simulink model "DEF_2SG"  (R2022b)
settings: Solver=FixedStepAuto  StartTime=0  StopTime=5  FixedStep=Ts  RelTol=1e-3
undefined symbols (not defined in the file or in its folder): ApparatusDiscreDamping, ApparatusPara, ApparatusPowerFlow, ApparatusType, OtherInputs, PowerFlow, Sbase, Ts, Vbase, Wbase, x_e, Ybase, Zbase
libraries: SimplusGT x6, spsGroundLib x5, spsThreePhaseSeriesRLCBranchLib x4, spsControlledCurrentSourceLib x3, spsCurrentMeasurementLib x3, spsVoltageMeasurementLib x3, spsThreePhaseParallelRLCBranchLib x2, spsabctoAlphaBetaZeroLib x2, spspowerguiLib x1
settings Model: Creator=yz34218  LastModifiedBy=yz34218

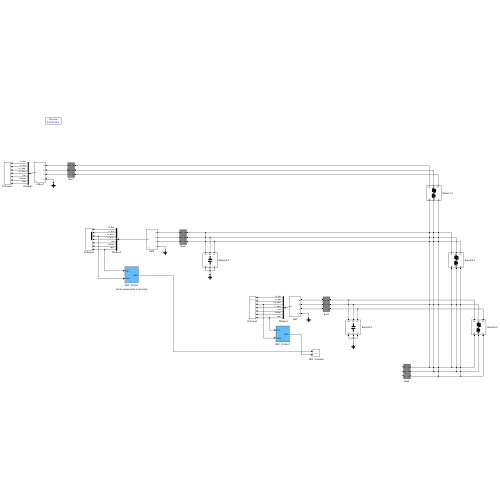
[thumbnail: Simulink's stored preview of the top-level diagram]
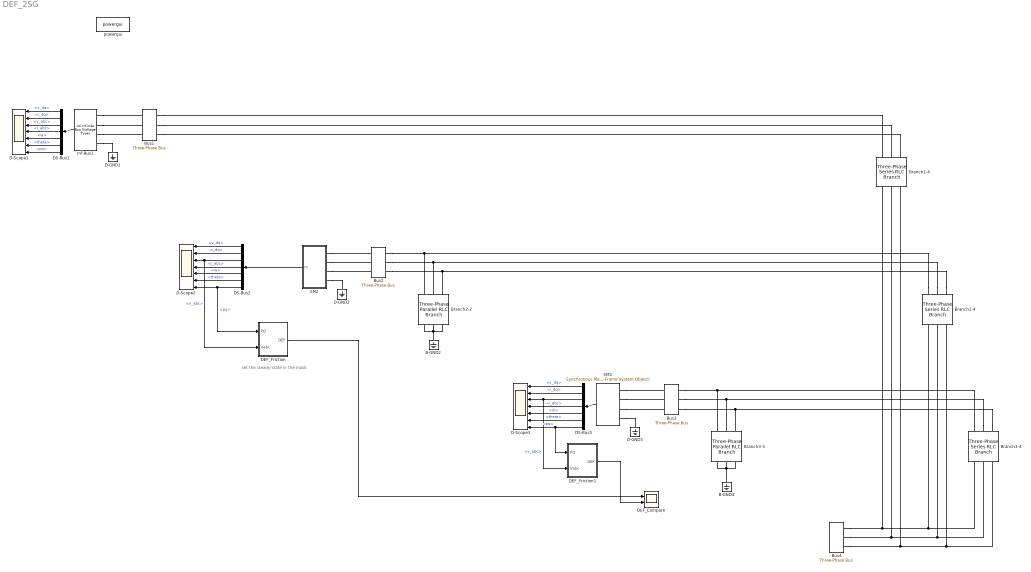
== system DEF_2SG ==
  note: set the steady-state in the mask
  B-GND2 : spsGroundLib/Ground  LConnTagsString=a
  B-GND4 : spsGroundLib/Ground  LConnTagsString=a
  Branch1-4 : spsThreePhaseSeriesRLCBranchLib/Three-Phase Series RLC Branch  LConnTagsString=A|B|C  RConnTagsString=A|B|C  BranchType=RL  Resistance=(0.1)*Zbase  Inductance=(1)*Zbase/Wbase  Capacitance=1e-6  Measurements=None
  Branch2-2 : spsThreePhaseParallelRLCBranchLib/Three-Phase Parallel RLC Branch  LConnTagsString=A|B|C  RConnTagsString=A|B|C  BranchType=C  Resistance=(Inf)*Zbase  Inductance=(Inf)*Zbase/Wbase  Capacitance=(0.3)*Ybase/Wbase  Measurements=None
  Branch2-4 : spsThreePhaseSeriesRLCBranchLib/Three-Phase Series RLC Branch  LConnTagsString=A|B|C  RConnTagsString=A|B|C  BranchType=RL  Resistance=(0.03)*Zbase  Inductance=(0.3)*Zbase/Wbase  Capacitance=1e-6  Measurements=None
  Branch3-3 : spsThreePhaseParallelRLCBranchLib/Three-Phase Parallel RLC Branch  LConnTagsString=A|B|C  RConnTagsString=A|B|C  BranchType=C  Resistance=(Inf)*Zbase  Inductance=(Inf)*Zbase/Wbase  Capacitance=(0.3)*Ybase/Wbase  Measurements=None
  Branch3-4 : spsThreePhaseSeriesRLCBranchLib/Three-Phase Series RLC Branch  LConnTagsString=A|B|C  RConnTagsString=A|B|C  BranchType=RL  Resistance=(0.03)*Zbase  Inductance=(0.3)*Zbase/Wbase  Capacitance=1e-6  Measurements=None
  Bus{1..4} (4 alike) : SimplusGT/Three-Phase Bus  Vbase=1  Sbase=1
  D-GND1 : spsGroundLib/Ground  LConnTagsString=a
  D-GND2 : spsGroundLib/Ground  LConnTagsString=a
  D-GND3 : spsGroundLib/Ground  LConnTagsString=a
  D-Scope1 : Scope  NumInputPorts=7
  D-Scope2 : Scope  NumInputPorts=7
  D-Scope3 : Scope  NumInputPorts=7
  DEF_Compare : Scope  NumInputPorts=2
  DEF_Friction : Subsystem  mask{PowerFlow_App=ApparatusPowerFlow{2}}
      mask prompts: PowerFlow_App "Power Flow"
  DEF_Friction1 : Subsystem  mask{PowerFlow_App=ApparatusPowerFlow{3}}
      mask prompts: PowerFlow_App "Power Flow"
  DS-Bus1 : BusSelector  OutputSignals=v_dq,i_dq,v_abc,i_abc,w,theta,pq
  DS-Bus2 : BusSelector  OutputSignals=v_dq,i_dq,v_abc,i_abc,w,theta,pq
  DS-Bus3 : BusSelector  OutputSignals=v_dq,i_dq,v_abc,i_abc,w,theta,pq
  Inf-Bus1 : SimplusGT/AC Infinite Bus (Voltage Type)  Ts=Ts  Sbase=Sbase  Vbase=Vbase  Wbase=Wbase  vd=PowerFlow{1}(3)  vq=0  theta0=PowerFlow{1}(4)  w=Wbase  R=1e-30
  SM2 : Subsystem  AncestorBlock=|  mask{Ts=Ts, Sbase=Sbase, Vbase=Vbase, Wbase=Wbase, ApparatusType=ApparatusType{2}, ApparatusPara=ApparatusPara{2}, PowerFlow=ApparatusPowerFlow{2}, x0=x_e{2}, OtherInputs=OtherInputs{2}, DiscreMethod=Hybrid Trapezoidal, EnableInsideModification=off, DiscreDampingFlag=on, DiscreDampingValue=ApparatusDiscreDamping{2}, LinearizationTimes=1, DirectFeedthrough=off}
      | SimplusGT/Synchronous Machine
      | (dq-Frame System Object)
      mask prompts: Ts "Ts (s), samping period"; Sbase "Sbase (VA), power base"; Vbase "Vbase (V), voltage base"; Wbase "Wbase (rad/s), frequency base"; ApparatusType "Apparatus type"; ApparatusPara "Apparatus parameters"; PowerFlow "Power flow paramters"; x0 "x0, initial states"; OtherInputs "Other inputs"; DiscreMethod "Discrerization method"; EnableInsideModification "Enable inside modification"; DiscreDampingFlag "Enable discretization damping"; DiscreDampingValue "Discretization damping value"; LinearizationTimes "Linearization times"; DirectFeedthrough "Direct feedthrough"
      mask init:
      | SimplusGT.Simulink.DeviceMaskInitialization(EnableInsideModification,DiscreDampingFlag);
      settings: LibrarySourceBlock=|
      | SimplusGT/Synchronous Machine
      | (dq-Frame System Object)
      mask TypeOptions DiscreMethod: Forward Euler | Hybrid Trapezoidal | Virtual Damping
      mask TypeOptions LinearizationTimes: 1 | 2
  SM3 : SimplusGT/Synchronous Machine (dq-Frame System Object)  Ts=Ts  Sbase=Sbase  Vbase=Vbase  Wbase=Wbase  ApparatusType=ApparatusType{3}  ApparatusPara=ApparatusPara{3}  PowerFlow=ApparatusPowerFlow{3}  x0=x_e{3}  OtherInputs=OtherInputs{3}  DiscreMethod=Hybrid Trapezoidal  EnableInsideModification=off  DiscreDampingFlag=on  DiscreDampingValue=ApparatusDiscreDamping{3}  LinearizationTimes=1  DirectFeedthrough=off
  powergui : spspowerguiLib/powergui  Priority=1  SimulationMode=Discrete  SampleTime=Ts  frequency=60  Iterations=50  frequencyindice=0  Pbase=100e6  ErrMax=1e-4  UnitsV=kV  UnitsW=MW  buscounter=0  FunctionMessages=off  echomessages=off  EnableUseOfTLC=off  CurrentSourceSwitches=off  DisableSnubberDevices=off  DisableRonSwitches=off  DisableVfSwitches=off  DisplayEquations=off  AutomaticDiscreteSolvers=off  SolverType=Tustin/Backward Euler (TBE)  Interpol=off  ExternalGateDelay=off  methode=off  Ts=100  x0status=blocks  SPID=on  SwTol=0  HookPort=off  NonlinearTolerance=1e-4  nMaxIteration=100  ContinueOnMaxIteration=off  RestoreLinks=warning  ResistiveCurrentMeasurement=off  Frange=[0:2:500]  Ylog=off  Xlog=on  ShowGrid=off  save=off  variable=ZData  structure=0  ZoomFFT=off  StartTime=0.0  cycles=1  DisplayStyle=1  fundamental=60  FreqAxis=off  MaxFrequency=1000  frequencyindicesteady=1  RmsSteady=1  display=off
  wires:
  Inf-Bus1/1 -> DS-Bus1/1
  DS-Bus1/1 -> D-Scope1/1  "<v_dq>"
  DS-Bus1/2 -> D-Scope1/2  "<i_dq>"
  DS-Bus1/3 -> D-Scope1/3  "<v_abc>"
  DS-Bus1/4 -> D-Scope1/4  "<i_abc>"
  DS-Bus1/5 -> D-Scope1/5  "<w>"
  DS-Bus1/6 -> D-Scope1/6  "<theta>"
  DS-Bus1/7 -> D-Scope1/7  "<pq>"
  SM2/1(m) -> DS-Bus2/1
  DS-Bus2/1 -> D-Scope2/1  "<v_dq>"
  DS-Bus2/2 -> D-Scope2/2  "<i_dq>"
  DS-Bus2/3 -> DEF_Friction/2(Vabc), D-Scope2/3  "<v_abc>"
  DS-Bus2/4 -> D-Scope2/4  "<i_abc>"
  DS-Bus2/5 -> D-Scope2/5  "<w>"
  DS-Bus2/6 -> D-Scope2/6  "<theta>"
  DS-Bus2/7 -> DEF_Friction/1(PQ), D-Scope2/7  "<pq>"
  SM3/1 -> DS-Bus3/1
  DS-Bus3/1 -> D-Scope3/1  "<v_dq>"
  DS-Bus3/2 -> D-Scope3/2  "<i_dq>"
  DS-Bus3/4 -> D-Scope3/4  "<i_abc>"
  DS-Bus3/5 -> D-Scope3/5  "<w>"
  DS-Bus3/6 -> D-Scope3/6  "<theta>"
  DS-Bus3/3 -> DEF_Friction1/2(Vabc), D-Scope3/3  "<v_abc>"
  DS-Bus3/7 -> DEF_Friction1/1(PQ), D-Scope3/7  "<pq>"
  DEF_Friction/1(DEF) -> DEF_Compare/1
  DEF_Friction1/1(DEF) -> DEF_Compare/2
  connections:
  Inf-Bus1/LConn4 -- D-GND1/LConn1
  SM2/LConn4 -- D-GND2/LConn1
  SM3/LConn4 -- D-GND3/LConn1
  Branch2-2/RConn1 -- Branch2-2/RConn2 -- Branch2-2/RConn3 -- B-GND2/LConn1
  Branch3-3/RConn2 -- Branch3-3/RConn1 -- B-GND4/LConn1 -- Branch3-3/RConn3
  Branch1-4/RConn1 -- Bus4/RConn1 -- Branch3-4/RConn1 -- Branch2-4/RConn1
  Branch1-4/RConn2 -- Bus4/RConn2 -- Branch3-4/RConn2 -- Branch2-4/RConn2
  Branch1-4/RConn3 -- Bus4/RConn3 -- Branch3-4/RConn3 -- Branch2-4/RConn3
  Bus1/RConn1 -- Branch1-4/LConn1
  Bus1/RConn2 -- Branch1-4/LConn2
  Bus1/RConn3 -- Branch1-4/LConn3
  Branch2-4/LConn1 -- Bus2/RConn1 -- Branch2-2/LConn1
  Branch2-4/LConn2 -- Bus2/RConn2 -- Branch2-2/LConn2
  Branch2-4/LConn3 -- Bus2/RConn3 -- Branch2-2/LConn3
  Branch3-4/LConn1 -- Bus3/RConn1 -- Branch3-3/LConn1
  Branch3-4/LConn2 -- Bus3/RConn2 -- Branch3-3/LConn2
  Branch3-4/LConn3 -- Bus3/RConn3 -- Branch3-3/LConn3
  Inf-Bus1/LConn1 -- Bus1/LConn1
  Inf-Bus1/LConn2 -- Bus1/LConn2
  Inf-Bus1/LConn3 -- Bus1/LConn3
  SM2/LConn1 -- Bus2/LConn1
  SM2/LConn2 -- Bus2/LConn2
  SM2/LConn3 -- Bus2/LConn3
  SM3/LConn1 -- Bus3/LConn1
  SM3/LConn2 -- Bus3/LConn2
  SM3/LConn3 -- Bus3/LConn3

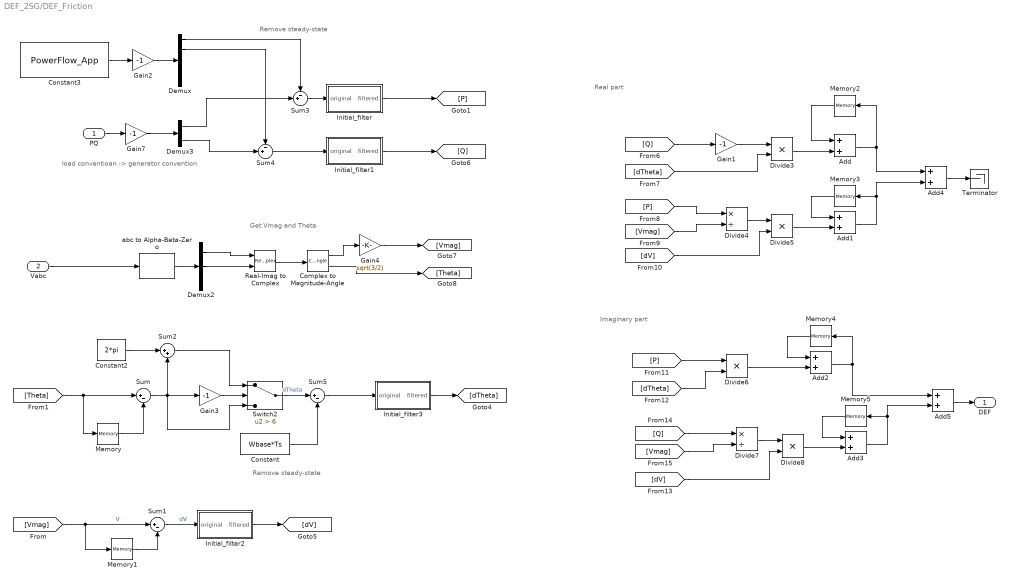
== system DEF_2SG/DEF_Friction ==
  note: Real part
  note: Imaginary part
  note: load conventioan -> generator convention
  note: Remove steady-state
  note: Remove steady-state
  note: Get Vmag and Theta
  PQ : Inport
  Vabc : Inport  Port=2
  Add{,1..5} (6 alike) : Sum
  Complex to Magnitude-Angle : ComplexToMagnitudeAngle
  Constant : Constant  Value=Wbase*Ts
  Constant2 : Constant  Value=2*pi
  Constant3 : Constant  Value=PowerFlow_App
  Demux : Demux  Outputs=5
  Demux2 : Demux  Outputs=3
  Demux3 : Demux  Outputs=2
  Divide{3,5..6,8} (4 alike) : Product  Inputs=**
  Divide4 : Product  Inputs=*/
  Divide7 : Product  Inputs=*/
  Gain{1..3,7} (4 alike) : Gain  Gain=-1
  Gain4 : Gain  Gain=sqrt(3/2)
  Initial_filter : Subsystem
  Initial_filter1 : Subsystem
  Initial_filter2 : Subsystem
  Initial_filter3 : Subsystem
  Memory{,1..5} (6 alike) : Memory
  Real-Imag to Complex : RealImagToComplex
  Sum : Sum  Inputs=|+-
  Sum1 : Sum  Inputs=|+-
  Sum2 : Sum  Inputs=|++
  Sum3 : Sum  Inputs=-+|
  Sum4 : Sum  Inputs=-+|
  Sum5 : Sum  Inputs=|+-
  Switch2 : Switch  Criteria=u2 > Threshold  Threshold=6  SaturateOnIntegerOverflow=off  InputSameDT=off
  Terminator : Terminator
  abc to Alpha-Beta-Zero : spsabctoAlphaBetaZeroLib/abc to Alpha-Beta-Zero
  DEF : Outport
  wires:
  [Q] -> Divide7/1
  [Vmag] -> Divide4/2
  Divide3/1 -> Add/2
  [P] -> Divide4/1
  [Q] -> Gain1/1
  Gain1/1 -> Divide3/1
  [dTheta] -> Divide3/2
  [dV] -> Divide5/2
  [P] -> Divide6/1
  Divide4/1 -> Divide5/1
  [dTheta] -> Divide6/2
  [dV] -> Divide8/2
  Divide7/1 -> Divide8/1
  [Vmag] -> Divide7/2
  Memory1/1 -> Sum1/2
  [Vmag] -> Memory1/1, Sum1/1  "V"
  Sum1/1 -> Initial_filter2/1(original)  "dV"
  [Theta] -> Sum/1, Memory/1
  Add/1 -> Memory2/1, Add4/1
  Memory2/1 -> Add/1
  Divide5/1 -> Add1/2
  Add1/1 -> Add4/2, Memory3/1
  Memory3/1 -> Add1/1
  Memory4/1 -> Add2/1
  Add2/1 -> Add5/1, Memory4/1
  Divide6/1 -> Add2/2
  Memory5/1 -> Add3/1
  Add3/1 -> Add5/2, Memory5/1
  Divide8/1 -> Add3/2
  Vabc/1 -> abc to Alpha-Beta-Zero/1
  abc to Alpha-Beta-Zero/1 -> Demux2/1
  Memory/1 -> Sum/2
  Sum/1 -> Gain3/1, Switch2/3, Sum2/2
  Sum2/1 -> Switch2/1
  Constant2/1 -> Sum2/1
  Gain3/1 -> Switch2/2
  Constant3/1 -> Gain2/1
  Sum3/1 -> Initial_filter/1(original)
  Demux/1 -> Sum3/1
  Sum4/1 -> Initial_filter1/1(original)
  Demux/2 -> Sum4/1
  Demux3/1 -> Sum3/2
  Demux3/2 -> Sum4/2
  PQ/1 -> Gain7/1
  Initial_filter/1(filtered) -> [P]
  Initial_filter1/1(filtered) -> [Q]
  Initial_filter2/1(filtered) -> [dV]
  Initial_filter3/1(filtered) -> [dTheta]
  Complex to Magnitude-Angle/2 -> [Theta]
  Gain4/1 -> [Vmag]
  Complex to Magnitude-Angle/1 -> Gain4/1
  Real-Imag to Complex/1 -> Complex to Magnitude-Angle/1
  Demux2/1 -> Real-Imag to Complex/1
  Demux2/2 -> Real-Imag to Complex/2
  Gain2/1 -> Demux/1
  Gain7/1 -> Demux3/1
  Switch2/1 -> Sum5/1  "dTheta"
  Sum5/1 -> Initial_filter3/1(original)
  Constant/1 -> Sum5/2
  Add5/1 -> DEF/1
  Add4/1 -> Terminator/1

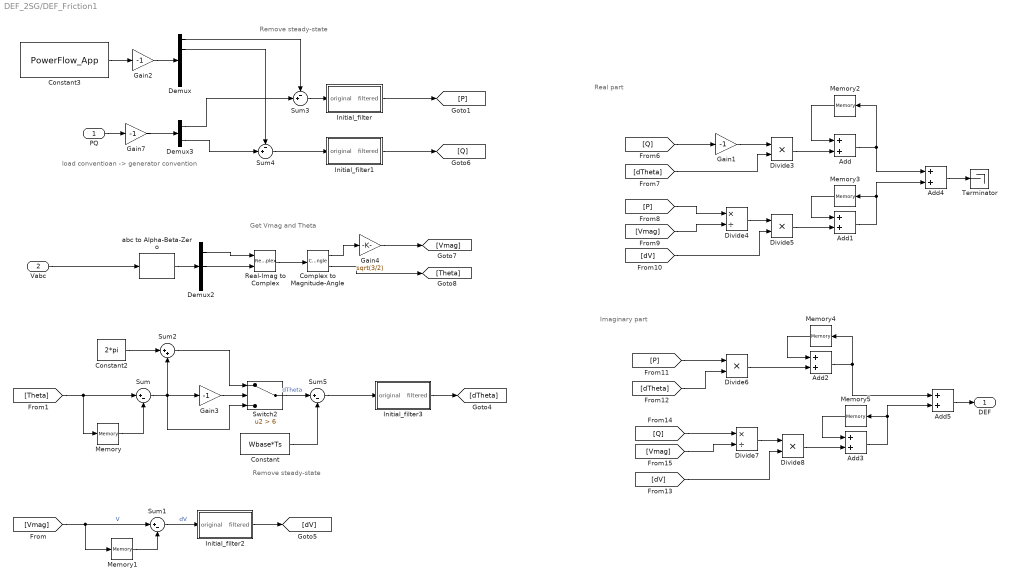
== system DEF_2SG/DEF_Friction1 ==
  note: Real part
  note: Imaginary part
  note: load conventioan -> generator convention
  note: Remove steady-state
  note: Remove steady-state
  note: Get Vmag and Theta
  PQ : Inport
  Vabc : Inport  Port=2
  Add{,1..5} (6 alike) : Sum
  Complex to Magnitude-Angle : ComplexToMagnitudeAngle
  Constant : Constant  Value=Wbase*Ts
  Constant2 : Constant  Value=2*pi
  Constant3 : Constant  Value=PowerFlow_App
  Demux : Demux  Outputs=5
  Demux2 : Demux  Outputs=3
  Demux3 : Demux  Outputs=2
  Divide{3,5..6,8} (4 alike) : Product  Inputs=**
  Divide4 : Product  Inputs=*/
  Divide7 : Product  Inputs=*/
  Gain{1..3,7} (4 alike) : Gain  Gain=-1
  Gain4 : Gain  Gain=sqrt(3/2)
  Initial_filter : Subsystem
  Initial_filter1 : Subsystem
  Initial_filter2 : Subsystem
  Initial_filter3 : Subsystem
  Memory{,1..5} (6 alike) : Memory
  Real-Imag to Complex : RealImagToComplex
  Sum : Sum  Inputs=|+-
  Sum1 : Sum  Inputs=|+-
  Sum2 : Sum  Inputs=|++
  Sum3 : Sum  Inputs=-+|
  Sum4 : Sum  Inputs=-+|
  Sum5 : Sum  Inputs=|+-
  Switch2 : Switch  Criteria=u2 > Threshold  Threshold=6  SaturateOnIntegerOverflow=off  InputSameDT=off
  Terminator : Terminator
  abc to Alpha-Beta-Zero : spsabctoAlphaBetaZeroLib/abc to Alpha-Beta-Zero
  DEF : Outport
  wires:
  [Q] -> Divide7/1
  [Vmag] -> Divide4/2
  Divide3/1 -> Add/2
  [P] -> Divide4/1
  [Q] -> Gain1/1
  Gain1/1 -> Divide3/1
  [dTheta] -> Divide3/2
  [dV] -> Divide5/2
  [P] -> Divide6/1
  Divide4/1 -> Divide5/1
  [dTheta] -> Divide6/2
  [dV] -> Divide8/2
  Divide7/1 -> Divide8/1
  [Vmag] -> Divide7/2
  Memory1/1 -> Sum1/2
  [Vmag] -> Memory1/1, Sum1/1  "V"
  Sum1/1 -> Initial_filter2/1(original)  "dV"
  [Theta] -> Sum/1, Memory/1
  Add/1 -> Memory2/1, Add4/1
  Memory2/1 -> Add/1
  Divide5/1 -> Add1/2
  Add1/1 -> Add4/2, Memory3/1
  Memory3/1 -> Add1/1
  Memory4/1 -> Add2/1
  Add2/1 -> Add5/1, Memory4/1
  Divide6/1 -> Add2/2
  Memory5/1 -> Add3/1
  Add3/1 -> Add5/2, Memory5/1
  Divide8/1 -> Add3/2
  Vabc/1 -> abc to Alpha-Beta-Zero/1
  abc to Alpha-Beta-Zero/1 -> Demux2/1
  Memory/1 -> Sum/2
  Sum/1 -> Gain3/1, Switch2/3, Sum2/2
  Sum2/1 -> Switch2/1
  Constant2/1 -> Sum2/1
  Gain3/1 -> Switch2/2
  Constant3/1 -> Gain2/1
  Sum3/1 -> Initial_filter/1(original)
  Demux/1 -> Sum3/1
  Sum4/1 -> Initial_filter1/1(original)
  Demux/2 -> Sum4/1
  Demux3/1 -> Sum3/2
  Demux3/2 -> Sum4/2
  PQ/1 -> Gain7/1
  Initial_filter/1(filtered) -> [P]
  Initial_filter1/1(filtered) -> [Q]
  Initial_filter2/1(filtered) -> [dV]
  Initial_filter3/1(filtered) -> [dTheta]
  Complex to Magnitude-Angle/2 -> [Theta]
  Gain4/1 -> [Vmag]
  Complex to Magnitude-Angle/1 -> Gain4/1
  Real-Imag to Complex/1 -> Complex to Magnitude-Angle/1
  Demux2/1 -> Real-Imag to Complex/1
  Demux2/2 -> Real-Imag to Complex/2
  Gain2/1 -> Demux/1
  Gain7/1 -> Demux3/1
  Switch2/1 -> Sum5/1  "dTheta"
  Sum5/1 -> Initial_filter3/1(original)
  Constant/1 -> Sum5/2
  Add5/1 -> DEF/1
  Add4/1 -> Terminator/1

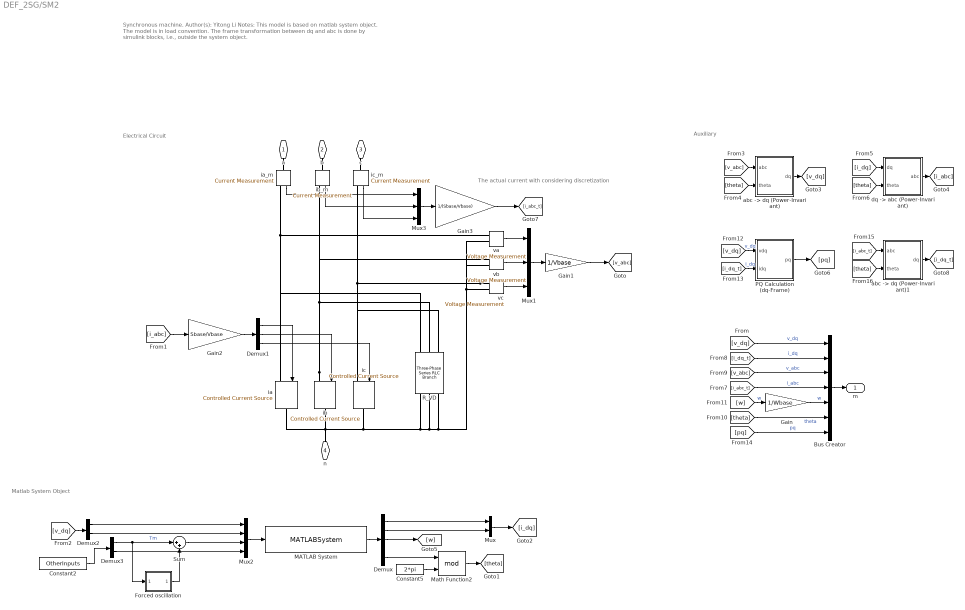
== system DEF_2SG/SM2 ==
  note: Electrical Circuit
  note: Auxiliary
  note: Matlab System Object
  note: Synchronous machine.
      |
      | Author(s): Yitong Li
      |
      | Notes:
      |
      | This model is based on matlab system object.
      |
      | The model is in load convention.
      |
      | The frame transformation between dq and abc is done by simulink blocks, i.e., outside the system object.
  note: The actual current with considering discretization
  Bus Creator : BusCreator  Inputs=7
  Constant2 : Constant  Value=OtherInputs
  Constant5 : Constant  Value=2*pi
  Demux : Demux  Outputs=5
  Demux1 : Demux  Outputs=3
  Demux2 : Demux  Outputs=2
  Demux3 : Demux  Outputs=2
  Forced oscillation : Subsystem
  Gain : Gain  Gain=1/Wbase
  Gain1 : Gain  Gain=1/Vbase
  Gain2 : Gain  Gain=Sbase/Vbase
  Gain3 : Gain  Gain=1/(Sbase/Vbase)
  MATLAB System : MATLABSystem  System=SimplusGT.Class.SynchronousMachine  Ts=Ts  Para=ApparatusPara  ApparatusType=ApparatusType  PowerFlow=PowerFlow  x0=x0  DiscreMethod=DiscreMethod  LinearizationTimes=LinearizationTimes  DirectFeedthrough=DirectFeedthrough  VirtualResistor=DiscreDampingFlag  EquiInitial=true  ElecPortIOs=[ 1, 2 ]  SimulateUsing=Code generation
      mask Type: SimplusGT.Class.SynchronousMachine
      mask Display:
      | disp('SynchronousMachine');
      | port_label('input',1,'u');
      | port_label('output',1,'y');
  Math Function2 : Math  Operator=mod  SignedPower=on
  Mux : Mux  Inputs=2
  Mux1 : Mux  Inputs=3
  Mux2 : Mux
  Mux3 : Mux  Inputs=3
  PQ Calculation (dq-Frame) : Subsystem  AncestorBlock=|
      | SimplusGT/PQ Calculation
      | (dq-Frame)
      settings: LibrarySourceBlock=|
      | SimplusGT/PQ Calculation
      | (dq-Frame)
  R_VD : spsThreePhaseSeriesRLCBranchLib/Three-Phase Series RLC Branch  LConnTagsString=A|B|C  RConnTagsString=A|B|C  BranchType=R  Resistance=DiscreDampingValue*Vbase^2/Sbase  Inductance=1e-3  Capacitance=1e-6  Measurements=None
  Sum : Sum  Inputs=|++
  "abc -> dq (Power-Invariant)" : Subsystem  AncestorBlock=|
      | SimplusGT/abc -> dq
      | (Power-Invariant)
      settings: LibrarySourceBlock=|
      | SimplusGT/abc -> dq
      | (Power-Invariant)
  "abc -> dq (Power-Invariant)1" : Subsystem  AncestorBlock=|
      | SimplusGT/abc -> dq
      | (Power-Invariant)
      settings: LibrarySourceBlock=|
      | SimplusGT/abc -> dq
      | (Power-Invariant)
  "dq -> abc (Power-Invariant)" : Subsystem  AncestorBlock=|
      | SimplusGT/dq -> abc
      | (Power-Invariant)
      settings: LibrarySourceBlock=|
      | SimplusGT/dq -> abc
      | (Power-Invariant)
  ia : spsControlledCurrentSourceLib/Controlled Current Source  Initialize=on  Source_Type=AC  Amplitude=0  Phase=0  Frequency=0  Measurements=None
  ia_m : spsCurrentMeasurementLib/Current Measurement  PhasorSimulation=off  OutputType=Complex  PSBequivalent=0
  ib : spsControlledCurrentSourceLib/Controlled Current Source  Initialize=on  Source_Type=AC  Amplitude=0  Phase=0  Frequency=0  Measurements=None
  ib_m : spsCurrentMeasurementLib/Current Measurement  PhasorSimulation=off  OutputType=Complex  PSBequivalent=0
  ic : spsControlledCurrentSourceLib/Controlled Current Source  Initialize=on  Source_Type=AC  Amplitude=0  Phase=0  Frequency=0  Measurements=None
  ic_m : spsCurrentMeasurementLib/Current Measurement  PhasorSimulation=off  OutputType=Complex  PSBequivalent=0
  va : spsVoltageMeasurementLib/Voltage Measurement  PhasorSimulation=off  OutputType=Complex  PSBequivalent=0
  vb : spsVoltageMeasurementLib/Voltage Measurement  PhasorSimulation=off  OutputType=Complex  PSBequivalent=0
  vc : spsVoltageMeasurementLib/Voltage Measurement  PhasorSimulation=off  OutputType=Complex  PSBequivalent=0
  a : PMIOPort  Side=Left
  b : PMIOPort  Port=2  Side=Left
  c : PMIOPort  Port=3  Side=Left
  n : PMIOPort  Port=4  Side=Left
  m : Outport
  wires:
  "abc -> dq (Power-Invariant)1"/1(dq) -> [i_dq_t]
  [theta] -> "abc -> dq (Power-Invariant)1"/2(theta)
  [i_abc_t] -> "abc -> dq (Power-Invariant)1"/1(abc)
  Gain3/1 -> [i_abc_t]
  Mux3/1 -> Gain3/1
  ic_m/1 -> Mux3/3
  ib_m/1 -> Mux3/2
  ia_m/1 -> Mux3/1
  Gain2/1 -> Demux1/1
  Gain1/1 -> [v_abc]
  [pq] -> Bus Creator/7  "pq"
  PQ Calculation (dq-Frame)/1(pq) -> [pq]
  [i_dq_t] -> PQ Calculation (dq-Frame)/2(idq)  "i_dq"
  [v_dq] -> PQ Calculation (dq-Frame)/1(vdq)  "v_dq"
  [i_abc] -> Gain2/1
  Demux3/2 -> Mux2/4
  Constant2/1 -> Demux3/1
  Mux1/1 -> Gain1/1
  Gain/1 -> Bus Creator/5  "w"
  Bus Creator/1 -> m/1
  [theta] -> Bus Creator/6  "theta"
  [w] -> Gain/1  "w"
  [i_abc_t] -> Bus Creator/4  "i_abc"
  [v_abc] -> Bus Creator/3  "v_abc"
  [i_dq_t] -> Bus Creator/2  "i_dq"
  [v_dq] -> Bus Creator/1  "v_dq"
  Math Function2/1 -> [theta]
  Constant5/1 -> Math Function2/2
  Demux/5 -> Math Function2/1
  Demux1/3 -> ic/1
  vc/1 -> Mux1/3
  MATLAB System/1 -> Demux/1
  Mux2/1 -> MATLAB System/1
  "dq -> abc (Power-Invariant)"/1(abc) -> [i_abc]
  [theta] -> "dq -> abc (Power-Invariant)"/2(theta)
  [i_dq] -> "dq -> abc (Power-Invariant)"/1(dq)
  "abc -> dq (Power-Invariant)"/1(dq) -> [v_dq]
  [theta] -> "abc -> dq (Power-Invariant)"/2(theta)
  [v_abc] -> "abc -> dq (Power-Invariant)"/1(abc)
  Demux2/2 -> Mux2/2
  Demux2/1 -> Mux2/1
  [v_dq] -> Demux2/1
  vb/1 -> Mux1/2
  va/1 -> Mux1/1
  Demux1/2 -> ib/1
  Demux1/1 -> ia/1
  Demux/3 -> [w]
  Mux/1 -> [i_dq]
  Demux/1 -> Mux/1
  Demux/2 -> Mux/2
  Demux3/1 -> Sum/1, Forced oscillation/1(Tm)  "Tm"
  Forced oscillation/1(Out1) -> Sum/2
  Sum/1 -> Mux2/3
  connections:
  ic_m/LConn1 -- c/RConn1
  ib_m/LConn1 -- b/RConn1
  ia_m/LConn1 -- a/RConn1
  ia_m/RConn1 -- ia/LConn1 -- R_VD/LConn1 -- va/LConn1
  vc/LConn1 -- ic_m/RConn1 -- ic/LConn1 -- R_VD/LConn3
  ib/LConn1 -- ib_m/RConn1 -- vb/LConn1 -- R_VD/LConn2
  ic/RConn1 -- n/RConn1 -- ib/RConn1 -- ia/RConn1 -- R_VD/RConn1 -- R_VD/RConn2 -- R_VD/RConn3 -- vc/LConn2 -- va/LConn2 -- vb/LConn2

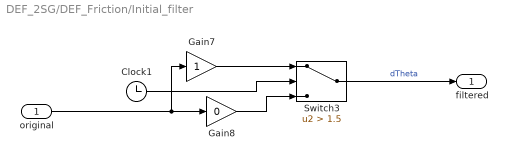
== system DEF_2SG/DEF_Friction/Initial_filter ==
  original : Inport
  Clock1 : Clock
  Gain7 : Gain
  Gain8 : Gain  Gain=0
  Switch3 : Switch  Criteria=u2 > Threshold  Threshold=1.5  SaturateOnIntegerOverflow=off  InputSameDT=off
  filtered : Outport
  wires:
  Switch3/1 -> filtered/1  "dTheta"
  original/1 -> Gain8/1, Gain7/1
  Gain7/1 -> Switch3/1
  Gain8/1 -> Switch3/3
  Clock1/1 -> Switch3/2

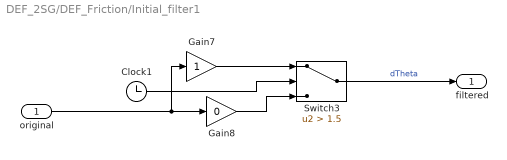
== system DEF_2SG/DEF_Friction/Initial_filter1 ==
  original : Inport
  Clock1 : Clock
  Gain7 : Gain
  Gain8 : Gain  Gain=0
  Switch3 : Switch  Criteria=u2 > Threshold  Threshold=1.5  SaturateOnIntegerOverflow=off  InputSameDT=off
  filtered : Outport
  wires:
  Switch3/1 -> filtered/1  "dTheta"
  original/1 -> Gain8/1, Gain7/1
  Gain7/1 -> Switch3/1
  Gain8/1 -> Switch3/3
  Clock1/1 -> Switch3/2

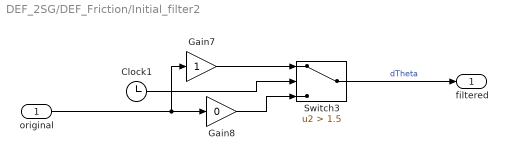
== system DEF_2SG/DEF_Friction/Initial_filter2 ==
  original : Inport
  Clock1 : Clock
  Gain7 : Gain
  Gain8 : Gain  Gain=0
  Switch3 : Switch  Criteria=u2 > Threshold  Threshold=1.5  SaturateOnIntegerOverflow=off  InputSameDT=off
  filtered : Outport
  wires:
  Switch3/1 -> filtered/1  "dTheta"
  original/1 -> Gain8/1, Gain7/1
  Gain7/1 -> Switch3/1
  Gain8/1 -> Switch3/3
  Clock1/1 -> Switch3/2

== system DEF_2SG/DEF_Friction/Initial_filter3 ==
  original : Inport
  Clock1 : Clock
  Gain7 : Gain
  Gain8 : Gain  Gain=0
  Switch3 : Switch  Criteria=u2 > Threshold  Threshold=1.5  SaturateOnIntegerOverflow=off  InputSameDT=off
  filtered : Outport
  wires:
  Switch3/1 -> filtered/1  "dTheta"
  original/1 -> Gain8/1, Gain7/1
  Gain7/1 -> Switch3/1
  Gain8/1 -> Switch3/3
  Clock1/1 -> Switch3/2

== system DEF_2SG/DEF_Friction1/Initial_filter ==
  original : Inport
  Clock1 : Clock
  Gain7 : Gain
  Gain8 : Gain  Gain=0
  Switch3 : Switch  Criteria=u2 > Threshold  Threshold=1.5  SaturateOnIntegerOverflow=off  InputSameDT=off
  filtered : Outport
  wires:
  Switch3/1 -> filtered/1  "dTheta"
  original/1 -> Gain8/1, Gain7/1
  Gain7/1 -> Switch3/1
  Gain8/1 -> Switch3/3
  Clock1/1 -> Switch3/2

== system DEF_2SG/DEF_Friction1/Initial_filter1 ==
  original : Inport
  Clock1 : Clock
  Gain7 : Gain
  Gain8 : Gain  Gain=0
  Switch3 : Switch  Criteria=u2 > Threshold  Threshold=1.5  SaturateOnIntegerOverflow=off  InputSameDT=off
  filtered : Outport
  wires:
  Switch3/1 -> filtered/1  "dTheta"
  original/1 -> Gain8/1, Gain7/1
  Gain7/1 -> Switch3/1
  Gain8/1 -> Switch3/3
  Clock1/1 -> Switch3/2

== system DEF_2SG/DEF_Friction1/Initial_filter2 ==
  original : Inport
  Clock1 : Clock
  Gain7 : Gain
  Gain8 : Gain  Gain=0
  Switch3 : Switch  Criteria=u2 > Threshold  Threshold=1.5  SaturateOnIntegerOverflow=off  InputSameDT=off
  filtered : Outport
  wires:
  Switch3/1 -> filtered/1  "dTheta"
  original/1 -> Gain8/1, Gain7/1
  Gain7/1 -> Switch3/1
  Gain8/1 -> Switch3/3
  Clock1/1 -> Switch3/2

== system DEF_2SG/DEF_Friction1/Initial_filter3 ==
  original : Inport
  Clock1 : Clock
  Gain7 : Gain
  Gain8 : Gain  Gain=0
  Switch3 : Switch  Criteria=u2 > Threshold  Threshold=1.5  SaturateOnIntegerOverflow=off  InputSameDT=off
  filtered : Outport
  wires:
  Switch3/1 -> filtered/1  "dTheta"
  original/1 -> Gain8/1, Gain7/1
  Gain7/1 -> Switch3/1
  Gain8/1 -> Switch3/3
  Clock1/1 -> Switch3/2

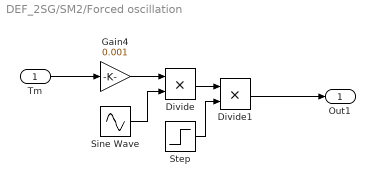
== system DEF_2SG/SM2/Forced oscillation ==
  Tm : Inport
  Divide : Product  Inputs=**
  Divide1 : Product  Inputs=**
  Gain4 : Gain  Gain=0.001
  Sine Wave : Sin  Frequency=2*pi*3  SampleTime=0
  Step : Step  Time=2  SampleTime=0
  Out1 : Outport
  wires:
  Gain4/1 -> Divide/1
  Divide1/1 -> Out1/1
  Divide/1 -> Divide1/1
  Step/1 -> Divide1/2
  Sine Wave/1 -> Divide/2
  Tm/1 -> Gain4/1

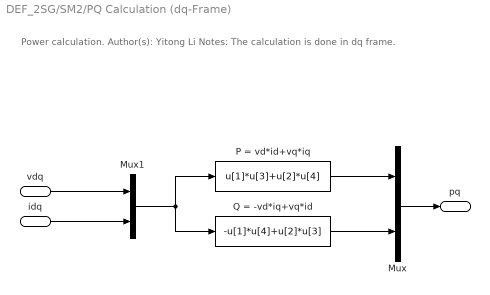
== system DEF_2SG/SM2/PQ Calculation (dq-Frame) ==
  note: Power calculation.
      |
      | Author(s): Yitong Li
      |
      | Notes:
      |
      | The calculation is done in dq frame.
  vdq : Inport
  idq : Inport  Port=2
  Mux : Mux  Inputs=2
  Mux1 : Mux  Inputs=2
  P = vd*id+vq*iq : Fcn  Expr=u[1]*u[3]+u[2]*u[4]
  Q = -vd*iq+vq*id : Fcn  Expr=-u[1]*u[4]+u[2]*u[3]
  pq : Outport
  wires:
  Mux/1 -> pq/1
  P = vd*id+vq*iq/1 -> Mux/1
  vdq/1 -> Mux1/1
  idq/1 -> Mux1/2
  Mux1/1 -> P = vd*id+vq*iq/1, Q = -vd*iq+vq*id/1
  Q = -vd*iq+vq*id/1 -> Mux/2

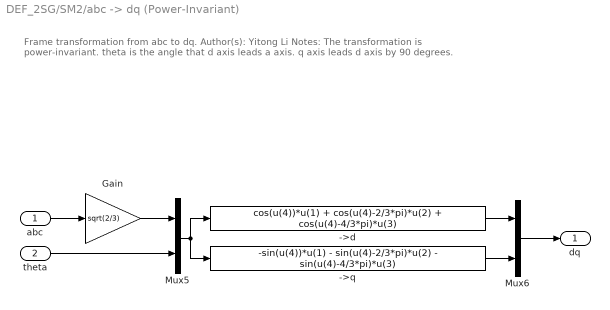
== system DEF_2SG/SM2/abc -> dq (Power-Invariant) ==
  note: Frame transformation from abc to dq.
      |
      | Author(s): Yitong Li
      |
      | Notes:
      |
      | The transformation is power-invariant.
      |
      | theta is the angle that d axis leads a axis.
      |
      | q axis leads d axis by 90 degrees.
  abc : Inport
  theta : Inport  Port=2
  ->d : Fcn  Expr=cos(u(4))*u(1) + cos(u(4)-2/3*pi)*u(2) + cos(u(4)-4/3*pi)*u(3)
  ->q : Fcn  Expr=-sin(u(4))*u(1) - sin(u(4)-2/3*pi)*u(2) - sin(u(4)-4/3*pi)*u(3)
  Gain : Gain  Gain=sqrt(2/3)
  Mux5 : Mux  Inputs=2
  Mux6 : Mux  Inputs=2
  dq : Outport
  wires:
  abc/1 -> Gain/1
  ->d/1 -> Mux6/1
  Gain/1 -> Mux5/1
  theta/1 -> Mux5/2
  ->q/1 -> Mux6/2
  Mux6/1 -> dq/1
  Mux5/1 -> ->d/1, ->q/1

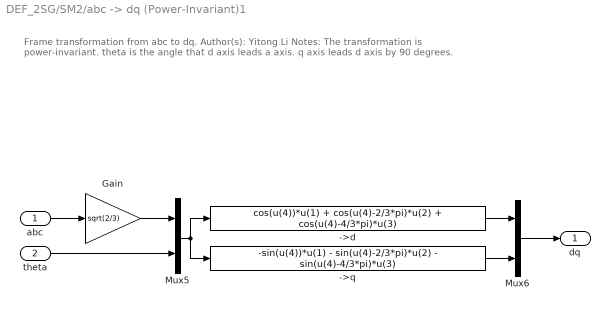
== system DEF_2SG/SM2/abc -> dq (Power-Invariant)1 ==
  note: Frame transformation from abc to dq.
      |
      | Author(s): Yitong Li
      |
      | Notes:
      |
      | The transformation is power-invariant.
      |
      | theta is the angle that d axis leads a axis.
      |
      | q axis leads d axis by 90 degrees.
  abc : Inport
  theta : Inport  Port=2
  ->d : Fcn  Expr=cos(u(4))*u(1) + cos(u(4)-2/3*pi)*u(2) + cos(u(4)-4/3*pi)*u(3)
  ->q : Fcn  Expr=-sin(u(4))*u(1) - sin(u(4)-2/3*pi)*u(2) - sin(u(4)-4/3*pi)*u(3)
  Gain : Gain  Gain=sqrt(2/3)
  Mux5 : Mux  Inputs=2
  Mux6 : Mux  Inputs=2
  dq : Outport
  wires:
  abc/1 -> Gain/1
  ->d/1 -> Mux6/1
  Gain/1 -> Mux5/1
  theta/1 -> Mux5/2
  ->q/1 -> Mux6/2
  Mux6/1 -> dq/1
  Mux5/1 -> ->d/1, ->q/1

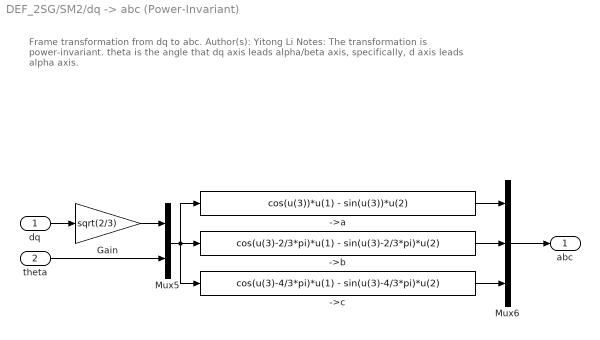
== system DEF_2SG/SM2/dq -> abc (Power-Invariant) ==
  note: Frame transformation from dq to abc.
      |
      | Author(s): Yitong Li
      |
      | Notes:
      |
      | The transformation is power-invariant.
      |
      | theta is the angle that dq axis leads alpha/beta axis, specifically, d axis leads alpha axis.
  dq : Inport
  theta : Inport  Port=2
  ->a : Fcn  Expr=cos(u(3))*u(1) - sin(u(3))*u(2)
  ->b : Fcn  Expr=cos(u(3)-2/3*pi)*u(1) - sin(u(3)-2/3*pi)*u(2)
  ->c : Fcn  Expr=cos(u(3)-4/3*pi)*u(1) - sin(u(3)-4/3*pi)*u(2)
  Gain : Gain  Gain=sqrt(2/3)
  Mux5 : Mux  Inputs=2
  Mux6 : Mux  Inputs=3
  abc : Outport
  wires:
  ->b/1 -> Mux6/2
  ->a/1 -> Mux6/1
  Gain/1 -> Mux5/1
  dq/1 -> Gain/1
  ->c/1 -> Mux6/3
  Mux6/1 -> abc/1
  Mux5/1 -> ->b/1, ->a/1, ->c/1
  theta/1 -> Mux5/2
